simulink model "P80s"  (R2015b)
settings: Solver=VariableStepAuto  StartTime=0.0  StopTime=5  RelTol=1e-3
settings Model: Creator=xmax1946  LastModifiedBy=xmax1946

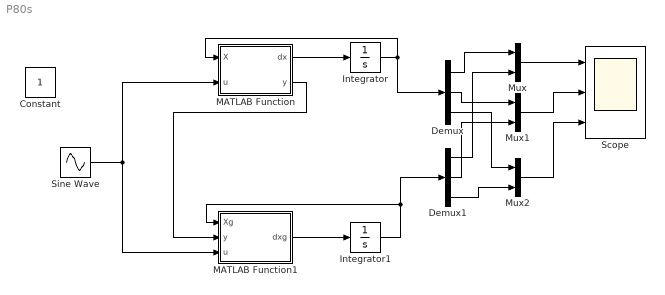
== system P80s ==
  Constant : Constant
  Demux : Demux  Outputs=3
  Demux1 : Demux  Outputs=3
  Integrator : Integrator  InitialCondition=[100;10;1]
  Integrator1 : Integrator  InitialCondition=[pi;pi;pi]
  MATLAB Function : MATLAB Function  TreatAsAtomicUnit=on
  MATLAB Function1 : MATLAB Function  TreatAsAtomicUnit=on
  Mux : Mux  Inputs=2
  Mux1 : Mux  Inputs=2
  Mux2 : Mux  Inputs=2
  Scope : Scope  NumInputPorts=3
  Sine Wave : Sin  Amplitude=10  SampleTime=0
  wires:
  MATLAB Function/1(dx) -> Integrator/1
  MATLAB Function1/1(dxg) -> Integrator1/1
  Integrator/1 -> MATLAB Function/1(X), Demux/1
  MATLAB Function/2(y) -> MATLAB Function1/2(y)
  Integrator1/1 -> Demux1/1, MATLAB Function1/1(Xg)
  Demux/1 -> Mux/1
  Demux1/1 -> Mux/2
  Demux/2 -> Mux1/1
  Demux1/2 -> Mux1/2
  Demux/3 -> Mux2/1
  Demux1/3 -> Mux2/2
  Mux/1 -> Scope/1
  Mux1/1 -> Scope/2
  Mux2/1 -> Scope/3
  Sine Wave/1 -> MATLAB Function1/3(u), MATLAB Function/2(u)

== matlab function P80s/MATLAB Function1 ==
  data: Xg input; y input; u input; dxg output
function dxg =fcn(Xg,y,u)
A=[-5,6,-7,1,6,-3,1;
    -3,1,-4,2,-5,7,1;
    0,0,-6,12,-14,6,1;
    0,0,0,6,-14,11,-8;
    0,0,0,7,-8,4,-8;
    0,0,0,0,0,3,-8;
    0,0,0,0,0,4,-5];
B=[3;2;1;0;0;0;0];
C=[1,-1,1,0,-1,1,-1];

L=[57.7467;0;-37.7467;-40.3067;0;0;0];
L=[58;0;-38;-40;0;0;0];

dxg=A*Xg+B*u+L*(y-C*Xg);

== matlab function P80s/MATLAB Function ==
  data: dx output; X input; y output; u input
function [dx,y]=fcn(X,u)
A=[-1,1,-2;0,-1,1;0,0,-1];
B=[1;0;1];
C=[1,0,0];

dx=A*X+B*u;
y=C*X;
